simulink model "Autoalign_system"  (Simulink 8.8)
settings: Solver=FixedStepAuto  StartTime=0.0  StopTime=inf  RelTol=1e-3  EnableMultiTasking=on
libraries: arduinolib x9
settings Model: Creator=Gebruiker  LastModifiedBy=Gebruiker  SimulationMode=external  ExtModeEnableFloating=off  ExtModeTrigDuration=2
settings DataIOCC: LimitDataPoints=off  SaveFormat=Dataset  SignalLoggingSaveFormat=Dataset
settings OptimizationCC: LifeSpan=auto  MaxStackSize=64
settings DebuggingCC: UnderspecifiedInitializationDetection=Simplified  MergeDetectMultiDrivingBlocksExec=error  ParameterTunabilityLossMsg=error  FcnCallInpInsideContextMsg=error  StateNameClashWarn=none  SFUnexpectedBacktrackingDiag=error  SFNoUnconditionalDefaultTransitionDiag=error  SFExecutionAtInitializationDiag=warning
settings HardwareCC: ProdBitPerInt=16  ProdBitPerPointer=16  ProdBitPerSizeT=16  ProdBitPerPtrDiffT=16  ProdIntDivRoundTo=Zero  ProdEndianess=LittleEndian  ProdWordSize=8  ProdHWDeviceType=Atmel->AVR
settings ModelReferenceCC: PropagateSignalLabelsOutOfModel=on
settings RTWCC: SystemTargetFile=ert.tlc  HardwareBoard=Arduino Mega 2560  TLCOptions=-aInlineSetEventsForThisBaseRateFcn=TLC_FALSE -aSuppressMultiTaskScheduler=TLC_FALSE -aRateBasedStepFcn=1  TemplateMakefile=ert_default_tmf  Description=Embedded Coder  GenerateReport=on  Toolchain=Arduino AVR  BuildConfiguration=Faster Runs  IncludeHyperlinkInReport=on  GenerateTraceInfo=on  GenerateTraceReport=on  GenerateTraceReportSl=on  GenerateTraceReportSf=on  GenerateTraceReportEml=on
settings MATStruct: className=codertarget.tools.BuildHook  argsTopModelOnly=[]  excludedModels=[]  includeReferencedModels=on  includeTopModel=on  enabled=on  UseCoderTarget=[1.0]  TargetHardware=Arduino Mega 2560  RTOS=Baremetal  Scheduler_interrupt_source=[0.0]  DataVersion=2016.02  IPAddress=codertarget.arduinobase.registry.getLoopbackIP;  Port=17725  Verbose=[1]  Configuration=Serial  COMPortBaud=921600  BuildAction=Build  Set_host_COM_port=Automatically  COM_port_number=1  Enable_overrun_detection=[0.0]  Digital_output_to_set_on_overrun=13  Analog_input_reference_voltage=[0.0]  Serial0_baud_rate=9600  Serial1_baud_rate=9600  Serial2_baud_rate=9600  Serial3_baud_rate=9600  SPI_clock_out_frequency=4000  SPI_mode=Mode 0 - Clock Polarity 0, Clock Phase 0  SPI_bitorder=MSB first  Disable_DHCP_Ethernet=[0.0]  Local_ip_address=192.168.0.20  Local_mac_address=DE:AD:BE:EF:FE:ED  Disable_DHCP_Wifi=[0.0]  Wifi_ip_address=192.168.1.20  Wifi_SSID=yourNetwork  Set_Wifi_Encryption=None  Wifi_WEP_key=D0D0DEADF00DABBADEAFBEADED  Wifi_WEP_key_index=0  Wifi_WPA_password=secretPassword  Enable_CustomServer=0  IP_address=184.106.153.149
settings CodeAppCC: IgnoreCustomStorageClasses=off  OperatorAnnotations=on  SimulinkDataObjDesc=on  SFDataObjDesc=on  MATLABFcnDesc=on  InsertBlockDesc=on  MATLABSourceComments=on
settings ERTTargetCC: TargetLangStandard=C99 (ISO)  MultiwordLength=2048  SupportContinuousTime=on  SupportVariableSizeSignals=on
settings ConfigComp: CovMetricSettings=dwe  CovHtmlReporting=off  CovSaveCumulativeToWorkspaceVar=off  CovSaveSingleToWorkspaceVar=off  CovExternalEMLEnable=on

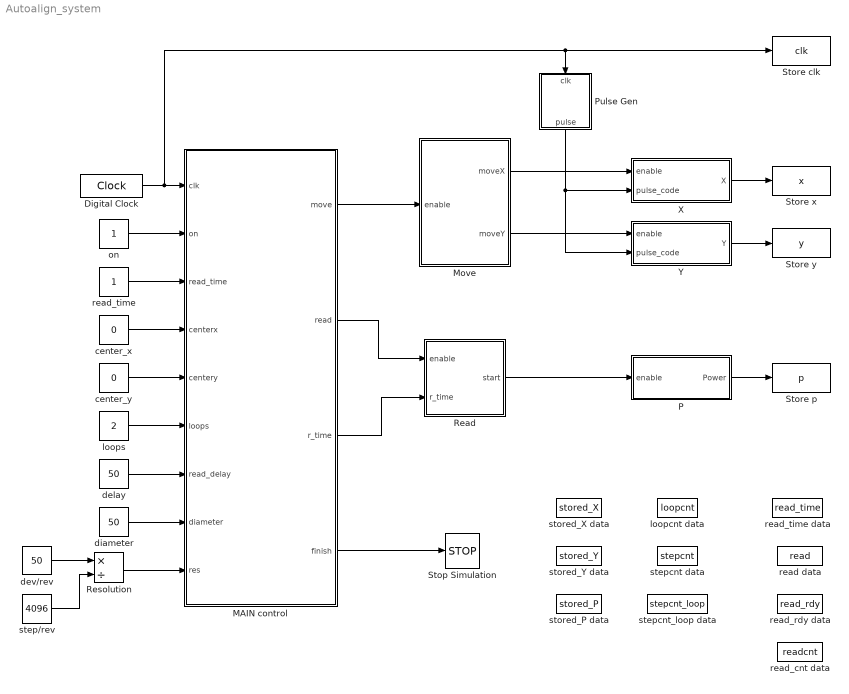
== system Autoalign_system ==
  Digital Clock : DigitalClock  SampleTime=.00125
  MAIN control : MATLAB Function  TreatAsAtomicUnit=on
  Move : MATLAB Function  TreatAsAtomicUnit=on
  P : Subsystem  Tag=p_block
  Pulse Gen : Subsystem  Tag=t_block
  Read : MATLAB Function  TreatAsAtomicUnit=on
  Resolution : Product  Inputs=*/
  Stop Simulation : Stop
  Store clk : ToWorkspace  VariableName=clk  SampleTime=-1
      settings: StopFcn=setappdata(0,'clk',clk);
  Store p : ToWorkspace  VariableName=p  SampleTime=-1
      settings: StopFcn=setappdata(0,'p_data',p);
  Store x : ToWorkspace  VariableName=x  SampleTime=-1
      settings: StopFcn=setappdata(0,'x_data',x);
  Store y : ToWorkspace  VariableName=y  SampleTime=-1
      settings: StopFcn=setappdata(0,'y_data',y);
  X : Subsystem  Tag=y_block
  Y : Subsystem  Tag=y_block
  center_x : Constant  Value=0
  center_y : Constant  Value=0
  delay : Constant  Value=50
  dev/rev : Constant  Value=50
  diameter : Constant  Value=50
  loopcnt data : DataStoreMemory  DataStoreName=loopcnt  ReadBeforeWriteMsg=warning  WriteAfterWriteMsg=warning  WriteAfterReadMsg=warning  InitialValue=1  ShowAdditionalParam=off  OutDataTypeStr=double
  loops : Constant  Value=2
  on : Constant
  read data : DataStoreMemory  DataStoreName=read  ReadBeforeWriteMsg=warning  WriteAfterWriteMsg=warning  WriteAfterReadMsg=warning  ShowAdditionalParam=off  OutDataTypeStr=double
  read_cnt data : DataStoreMemory  DataStoreName=readcnt  ReadBeforeWriteMsg=warning  WriteAfterWriteMsg=warning  WriteAfterReadMsg=warning  ShowAdditionalParam=off  OutDataTypeStr=double
  read_rdy data : DataStoreMemory  DataStoreName=read_rdy  ReadBeforeWriteMsg=warning  WriteAfterWriteMsg=warning  WriteAfterReadMsg=warning  ShowAdditionalParam=off  OutDataTypeStr=double
  read_time : Constant
  read_time data : DataStoreMemory  DataStoreName=read_time  ReadBeforeWriteMsg=warning  WriteAfterWriteMsg=warning  WriteAfterReadMsg=warning  ShowAdditionalParam=off  OutDataTypeStr=double
  step/rev : Constant  Value=4096
  stepcnt data : DataStoreMemory  DataStoreName=stepcnt  ReadBeforeWriteMsg=warning  WriteAfterWriteMsg=warning  WriteAfterReadMsg=warning  ShowAdditionalParam=off  OutDataTypeStr=double
  stepcnt_loop data : DataStoreMemory  DataStoreName=stepcnt_loop  ReadBeforeWriteMsg=warning  WriteAfterWriteMsg=warning  WriteAfterReadMsg=warning  ShowAdditionalParam=off  OutDataTypeStr=double
  stored_P data : DataStoreMemory  DataStoreName=stored_P  ReadBeforeWriteMsg=warning  WriteAfterWriteMsg=warning  WriteAfterReadMsg=warning  ShowAdditionalParam=off  OutDataTypeStr=double
  stored_X data : DataStoreMemory  DataStoreName=stored_X  ReadBeforeWriteMsg=warning  WriteAfterWriteMsg=warning  WriteAfterReadMsg=warning  ShowAdditionalParam=off  OutDataTypeStr=double
  stored_Y data : DataStoreMemory  DataStoreName=stored_Y  ReadBeforeWriteMsg=warning  WriteAfterWriteMsg=warning  WriteAfterReadMsg=warning  ShowAdditionalParam=off  OutDataTypeStr=double
  wires:
  on/1 -> MAIN control/2(on)
  loops/1 -> MAIN control/6(loops)
  delay/1 -> MAIN control/7(read_delay)
  diameter/1 -> MAIN control/8(diameter)
  Read/1(start) -> P/1(enable)
  MAIN control/1(move) -> Move/1(enable)
  MAIN control/2(read) -> Read/1(enable)
  Move/1(moveX) -> X/1(enable)
  Move/2(moveY) -> Y/1(enable)
  Pulse Gen/1(pulse) -> X/2(pulse_code), Y/2(pulse_code)
  Y/1(Y) -> Store y/1
  P/1(Power) -> Store p/1
  X/1(X) -> Store x/1
  Digital Clock/1 -> Store clk/1, Pulse Gen/1(clk), MAIN control/1(clk)
  center_x/1 -> MAIN control/4(centerx)
  center_y/1 -> MAIN control/5(centery)
  MAIN control/4(finish) -> Stop Simulation/1
  dev/rev/1 -> Resolution/1
  step/rev/1 -> Resolution/2
  Resolution/1 -> MAIN control/9(res)
  read_time/1 -> MAIN control/3(read_time)
  MAIN control/3(r_time) -> Read/2(r_time)

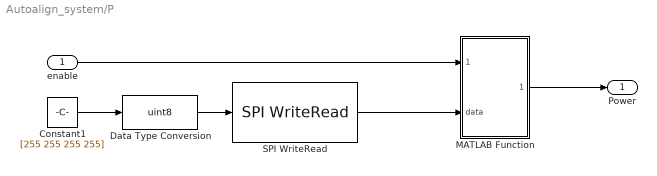
== system Autoalign_system/P ==
  enable : Inport
  Constant1 : Constant  Value=[255 255 255 255]
  Data Type Conversion : DataTypeConversion  OutDataTypeStr=uint8
  MATLAB Function : MATLAB Function  TreatAsAtomicUnit=on
  SPI WriteRead : arduinolib/SPI WriteRead  slaveSelectPin_=44  blockPlatform=arduino
  Power : Outport
  wires:
  Constant1/1 -> Data Type Conversion/1
  Data Type Conversion/1 -> SPI WriteRead/1
  SPI WriteRead/1 -> MATLAB Function/2(data)
  MATLAB Function/1(power) -> Power/1
  enable/1 -> MATLAB Function/1(enable)

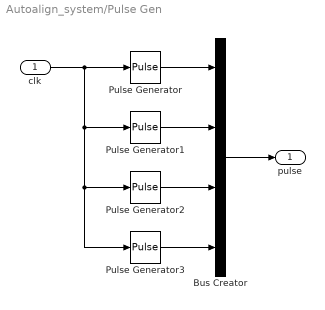
== system Autoalign_system/Pulse Gen ==
  clk : Inport
  Bus Creator : BusCreator  Inputs=4
  Pulse Generator : DiscretePulseGenerator  TimeSource=Use external signal  Period=8  PulseWidth=3
  Pulse Generator1 : DiscretePulseGenerator  TimeSource=Use external signal  Period=8  PulseWidth=3  PhaseDelay=2
  Pulse Generator2 : DiscretePulseGenerator  TimeSource=Use external signal  Period=8  PulseWidth=3  PhaseDelay=4
  Pulse Generator3 : DiscretePulseGenerator  TimeSource=Use external signal  Period=8  PulseWidth=3  PhaseDelay=6
  pulse : Outport
  wires:
  clk/1 -> Pulse Generator1/1, Pulse Generator2/1, Pulse Generator3/1, Pulse Generator/1
  Pulse Generator3/1 -> Bus Creator/4
  Pulse Generator1/1 -> Bus Creator/2
  Pulse Generator/1 -> Bus Creator/1
  Bus Creator/1 -> pulse/1
  Pulse Generator2/1 -> Bus Creator/3

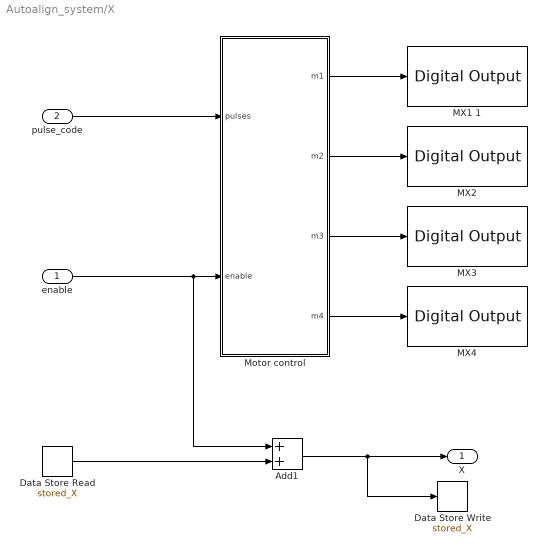
== system Autoalign_system/X ==
  enable : Inport
  pulse_code : Inport  Port=2
  Add1 : Sum
  Data Store Read : DataStoreRead  DataStoreName=stored_X
  Data Store Write : DataStoreWrite  DataStoreName=stored_X
  MX1 1 : arduinolib/Digital Output  pinNumber=2  blockPlatform=arduino
  MX2 : arduinolib/Digital Output  pinNumber=3  blockPlatform=arduino
  MX3 : arduinolib/Digital Output  pinNumber=4  blockPlatform=arduino
  MX4 : arduinolib/Digital Output  pinNumber=5  blockPlatform=arduino
  Motor control : MATLAB Function  TreatAsAtomicUnit=on
  X : Outport
  wires:
  pulse_code/1 -> Motor control/1(pulses)
  Motor control/4(m4) -> MX4/1
  Motor control/3(m3) -> MX3/1
  Motor control/2(m2) -> MX2/1
  Motor control/1(m1) -> MX1 1/1
  enable/1 -> Add1/1, Motor control/2(enable)
  Add1/1 -> Data Store Write/1, X/1
  Data Store Read/1 -> Add1/2

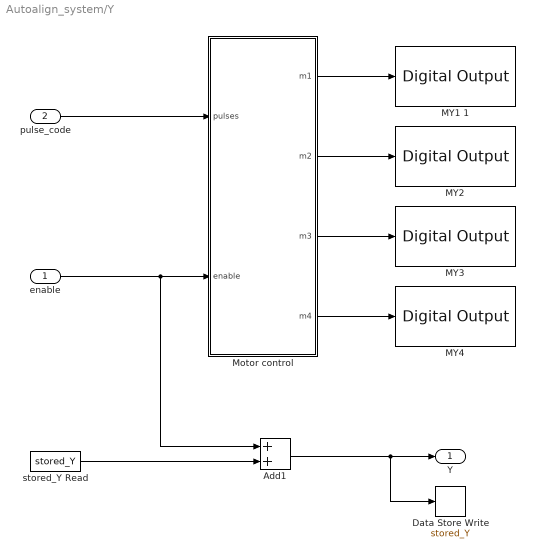
== system Autoalign_system/Y ==
  enable : Inport
  pulse_code : Inport  Port=2
  Add1 : Sum
  Data Store Write : DataStoreWrite  DataStoreName=stored_Y
  MY1 1 : arduinolib/Digital Output  pinNumber=8  blockPlatform=arduino
  MY2 : arduinolib/Digital Output  pinNumber=9  blockPlatform=arduino
  MY3 : arduinolib/Digital Output  pinNumber=10  blockPlatform=arduino
  MY4 : arduinolib/Digital Output  pinNumber=11  blockPlatform=arduino
  Motor control : MATLAB Function  TreatAsAtomicUnit=on
  stored_Y Read : DataStoreRead  DataStoreName=stored_Y
  Y : Outport
  wires:
  pulse_code/1 -> Motor control/1(pulses)
  Motor control/4(m4) -> MY4/1
  Motor control/3(m3) -> MY3/1
  Motor control/2(m2) -> MY2/1
  Motor control/1(m1) -> MY1 1/1
  enable/1 -> Add1/1, Motor control/2(enable)
  Add1/1 -> Data Store Write/1, Y/1
  stored_Y Read/1 -> Add1/2

== matlab function Read ==
  data: enable input double; start output double; read_rdy data_store_memory double; read_time data_store_memory double; r_time input double
function start = READ(enable,r_time)
global read_rdy;
global read_time;
if enable==1
    if read_rdy==0
        if read_time<=r_time
            start=0;
            read_rdy=0;
            read_time=read_time+1;
        else
            start=1;
            read_rdy=1;
            read_time=0;
        end
    else
        start=0;
        read_rdy=0;
    end
else
    start=0;
    read_rdy=0;
end

== matlab function MAIN control ==
  data: clk input double; on input double; read_time input double; centerx input double; centery input double; move output double; loops input double; read_delay input double; diameter input double; read output double; r_time output double; finish output double; stepcnt data_store_memory double; loopcnt data_store_memory double; stepcnt_loop data_store_memory double; read_rdy data_store_memory double; readcnt data_store_memory double; res input double
function [move,read,r_time,finish] = MAIN(clk,on,read_time,centerx,centery,loops,read_delay,diameter,res)
% variable declaration
global stepcnt;
global loopcnt;
global stepcnt_loop;
global read_rdy;
global readcnt;
r_time=read_time;
% initialization
if clk==0
    stepcnt=0;
    loopcnt=1;
    stepcnt_loop=(2*loopcnt-1)*diameter/((2*loops-1)*res);
end

% main code
if on==1
    % system is active
    if readcnt==read_delay
        % read active
        move=0;
        if read_rdy==1
            % read is ready
            read=0;
            readcnt=0;
        else
            % read not ready
            read=1;
        end
        finish=0;
    else
        % move
        read=0;
        readcnt=readcnt+1;
        if stepcnt<=stepcnt_loop
            % 1st part (move right)
            move=1;
            stepcnt=stepcnt+1;
            finish=0;
        elseif stepcnt<stepcnt_loop*2
            % 2nd part (move up)
            move=2;
            stepcnt=stepcnt+1;
            finish=0;
        elseif stepcnt<stepcnt_loop*3
            % 3rd part (move left)
            move=3;
            stepcnt=stepcnt+1;
            finish=0;
        elseif stepcnt<stepcnt_loop*4
            % 4th part (move down)
            move=4;
            stepcnt=stepcnt+1;
            finish=0;
        elseif loopcnt<loops
            if stepcnt<diameter/((2*loops-1)*res)+stepcnt_loop*4
                % 5th part (move to new loop)
                move=5;
                stepcnt=stepcnt+1;
                finish=0;
            else
                % number of steps is reached, new loop started
                move=0;
                stepcnt=0;
                loopcnt=loopcnt+1;
                stepcnt_loop=(2*loopcnt-1)*diameter/((2*loops-1)*res);
                finish=0;
            end
        else
            % number of loops is reached, simulation will stop
            move=0;
            stepcnt=0;
            finish=1;
        end
    end
elseif on==2
    % system is paused, simulation can continue any time
    move=0;
    read=0;
    finish=0;
else
    % system is turned off, simulation will stop
    move=0;
    read=0;
    finish=1;
end

== matlab function P/MATLAB Function ==
  data: enable input double; power output double; data input double; stored_P data_store_memory double
function power = CALCP(enable, data)
% variable declaration
global stored_P;

% main code
if enable==1
    % calculate new power
    powbi1=[fliplr(de2bi(data(1,1),8)) fliplr(de2bi(data(1,2),8)) fliplr(de2bi(data(1,3),8)) fliplr(de2bi(data(1,4),8))];
    pow0=bi2de(fliplr(powbi1(1,4:32)));
    pow1=double(pow0)./167772150 - 0.0015;
    stored_P=double(pow1);
end
% update power
power=stored_P;

== matlab function Move ==
  data: enable input double; moveX output double; moveY output double
function [moveX,moveY] = MOVE(enable)
switch enable
    case 1
        moveX=1;
        moveY=0;
    case 2
        moveX=0;
        moveY=1;
    case 3
        moveX=-1;
        moveY=0;
    case 4
        moveX=0;
        moveY=-1;
    case 5
        moveX=-1;
        moveY=-1;
    otherwise
        moveX=0;
        moveY=0;
end

== matlab function X/Motor control ==
  data: pulses input double; enable input double; m1 output double; m2 output double; m3 output double; m4 output double
function [m1,m2,m3,m4] = MOTOR(pulses,enable)
switch enable
    case 1
        m1=pulses(1);
        m2=pulses(2);
        m3=pulses(3);
        m4=pulses(4);
    case -1
        m1=pulses(4);
        m2=pulses(3);
        m3=pulses(2);
        m4=pulses(1);
    otherwise
        m1=0;
        m2=0;
        m3=0;
        m4=0;
end

== matlab function Y/Motor control ==
  data: pulses input double; enable input double; m1 output double; m2 output double; m3 output double; m4 output double
function [m1,m2,m3,m4] = MOTOR(pulses,enable)
switch enable
    case 1
        m1=pulses(1);
        m2=pulses(2);
        m3=pulses(3);
        m4=pulses(4);
    case -1
        m1=pulses(4);
        m2=pulses(3);
        m3=pulses(2);
        m4=pulses(1);
    otherwise
        m1=0;
        m2=0;
        m3=0;
        m4=0;
end
